simulink model "ModeSelectWithDebounce"  (R2018a)
settings: Solver=FixedStepDiscrete  StartTime=0.0  StopTime=inf  FixedStep=.01  RelTol=1e-3
libraries: simulink x2, CustomLibrary x2
settings Model: SimulationMode=external  ExtModeTrigDuration=2  Creator=jonathancoulter  LastModifiedBy=jonathancoulter
settings OptimizationCC: UseFloatMulNetSlope=on  PassReuseOutputArgsThreshold=0  EfficientFloat2IntCast=on  MaxStackSize=64
settings DebuggingCC: ParameterTunabilityLossMsg=error
settings HardwareCC: ProdBitPerInt=16  ProdBitPerPointer=16  ProdBitPerSizeT=16  ProdBitPerPtrDiffT=16  ProdLargestAtomicFloat=None  ProdWordSize=8  ProdHWDeviceType=Atmel->AVR  UseEmbeddedCoderFeatures=off
settings ModelReferenceCC: ModelReferenceMinAlgLoopOccurrences=on
settings SFSimCC: MATLABDynamicMemAlloc=off
settings RTWCC: SystemTargetFile=ert.tlc  HardwareBoard=Arduino Mega 2560  TLCOptions=-aInlineSetEventsForThisBaseRateFcn=TLC_FALSE -aSuppressMultiTaskScheduler=TLC_FALSE -aRateBasedStepFcn=1  TemplateMakefile=ert_default_tmf  Toolchain=Arduino AVR  BuildConfiguration=Faster Runs
settings CodeAppCC: ForceParamTrailComments=on  OperatorAnnotations=on  StateflowObjectComments=on  MATLABSourceComments=on
settings ERTTargetCC: ERTCustomFileBanners=off  SupportContinuousTime=on  SupportNonInlinedSFcns=on  RemoveResetFunc=off  SupportVariableSizeSignals=on  ModelStepFunctionPrototypeControlCompliant=off

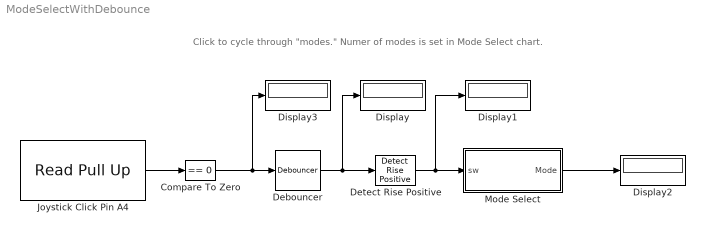
== system ModeSelectWithDebounce ==
  note: Click to cycle through "modes." Numer of modes is set in Mode Select chart.
  Compare To Zero : simulink/Logic and Bit Operations/Compare To Zero  relop===  OutDataTypeStr=boolean
  Debouncer : CustomLibrary/Debouncer
      settings: SourceProductName=Custom Blocks
  Detect Rise Positive : simulink/Logic and Bit Operations/Detect Rise Positive  vinit=0  OutDataTypeStr=boolean
  Display{,1..3} (4 alike) : Display
  Joystick Click Pin A4 : CustomLibrary/Read Pull Up  pinNumberMask=58  SampleTimeMask=0.1
      settings: SourceProductName=Custom Blocks
  Mode Select : Stateflow chart  TreatAsAtomicUnit=on
  wires:
  Debouncer/1 -> Display/1, Detect Rise Positive/1
  Detect Rise Positive/1 -> Display1/1, Mode Select/1(sw)
  Joystick Click Pin A4/1 -> Compare To Zero/1
  Compare To Zero/1 -> Debouncer/1, Display3/1
  Mode Select/1(Mode) -> Display2/1

== stateflow chart ModeSelectWithDebounce/Mode Select ==
  state Off
    en:
    Mode = 0;
  state Next_Mode
    en:
    Mode = Mode + 1;
  (default) -> Off
  Off -> Next_Mode : [sw == true]
  Next_Mode -> Off [order 2] : [sw == true]
  Next_Mode -> Next_Mode [order 1] : before(750, msec)
      | [sw == true && Mode < 10]
  data: sw input boolean; Mode output uint8
